simulink model "filtro2_fir_sim_r2015a"  (Simulink 8.5)
settings: Solver=FixedStepDiscrete  SolverMode=SingleTasking  StartTime=0.0  StopTime=1  RelTol=1e-3
values from neighbouring files (symbols this model uses):
  fa = 10000    [filtro2_fir.m]    (also in filtro2_iir.m)
undefined symbols (not defined in the file or in its folder): Ta
libraries: dspsrcs4 x4, dsparch4 x1
settings Model: Creator=vini  LastModifiedBy=vinicius.ls  CovMetricSettings=dwe  CovHtmlReporting=off  covSaveCumulativeToWorkspaceVar=off  CovSaveSingleToWorkspaceVar=off  CovExternalEMLEnable=on
settings DataIOCC: LimitDataPoints=off  SaveFormat=Dataset  SignalLoggingSaveFormat=Dataset
settings OptimizationCC: BlockReduction=off  ConditionallyExecuteInputs=off  InlineParams=on  ExpressionDepthLimit=128
settings DebuggingCC: AlgebraicLoopMsg=error  UnderspecifiedInitializationDetection=Simplified  MergeDetectMultiDrivingBlocksExec=error  FcnCallInpInsideContextMsg=EnableAllAsError  StateNameClashWarn=none  SFUnexpectedBacktrackingDiag=error  SFNoUnconditionalDefaultTransitionDiag=error
settings HardwareCC: ProdHWDeviceType=ASIC/FPGA->ASIC/FPGA  ProdEqTarget=off
settings ModelReferenceCC: PropagateSignalLabelsOutOfModel=on
settings SFSimCC: SimUseLocalCustomCode=on
settings RTWCC: RTWUseLocalCustomCode=on
settings GRTTargetCC: TargetLangStandard=C99 (ISO)  GeneratePreprocessorConditionals=Use local settings  CombineOutputUpdateFcns=on  GRTInterface=off

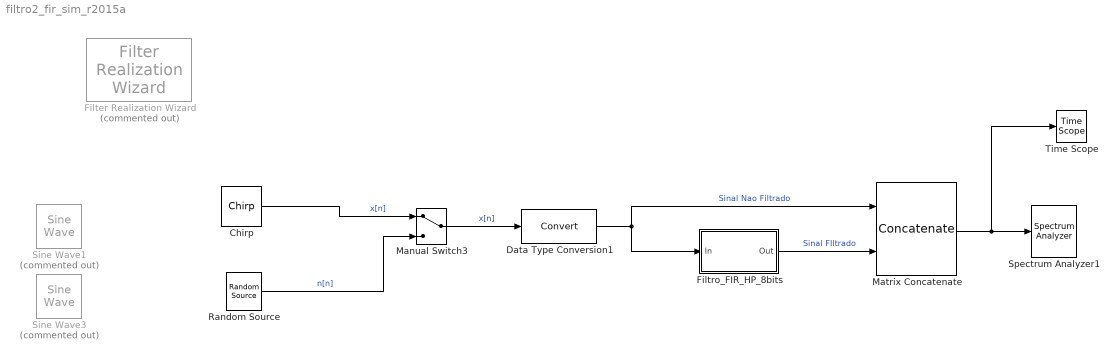
== system filtro2_fir_sim_r2015a ==
  Chirp : dspsrcs4/Chirp  sweep=Linear  mode=Unidirectional  f0=0  f1=fa/2  t1=1  Tsweep=1  phase=0  Ts=Ta  spf=spf  datatype=Double
  Data Type Conversion1 : DataTypeConversion
  Filter Realization Wizard : dsparch4/Filter Realization Wizard  Commented=on
  Filtro_FIR_HP_8bits : Subsystem  Tag=BlockMethodSubSystem
  Manual Switch3 : ManualSwitch
  Matrix Concatenate : Concatenate  Mode=Multidimensional array  ConcatenateDimension=2
  Random Source : dspsrcs4/Random Source  SrcType=Uniform  NormMethod=Ziggurat  CltLength=12  MinVal=-1  MaxVal=1  MeanVal=0  VarVal=1  RepMode=Not repeatable  rawSeed=1  IsInherit=off  SampMode=Discrete  SampTime=Ta  SampFrame=spf  DataType=Single  OutComplex=Real
  Sine Wave1 : dspsrcs4/Sine Wave  Commented=on  Amplitude=1  Frequency=100  Phase=0  SampleMode=Discrete  OutComplex=Real  CompMethod=Trigonometric fcn  TableSize=Speed  SampleTime=1/8000  SamplesPerFrame=1  ResetState=Restart at time zero  dataType=double  wordLen=16  udDataType=sfix(16)  fracBitsMode=Best precision  numFracBits=15  OutDataTypeStr=double  LastOutDataTypeStr=double
  Sine Wave3 : dspsrcs4/Sine Wave  Commented=on  Amplitude=1  Frequency=100  Phase=0  SampleMode=Discrete  OutComplex=Real  CompMethod=Trigonometric fcn  TableSize=Speed  SampleTime=1/8000  SamplesPerFrame=1  ResetState=Restart at time zero  dataType=double  wordLen=16  udDataType=sfix(16)  fracBitsMode=Best precision  numFracBits=15  OutDataTypeStr=double  LastOutDataTypeStr=double
  Spectrum Analyzer1 : SpectrumAnalyzer
  Time Scope : TimeScope  DefaultConfigurationName=spbscopes.TimeScopeBlockCfg
  wires:
  Data Type Conversion1/1 -> Filtro_FIR_HP_8bits/1(In), Matrix Concatenate/1  "Sinal Nao Filtrado"
  Matrix Concatenate/1 -> Time Scope/1, Spectrum Analyzer1/1
  Filtro_FIR_HP_8bits/1(Out) -> Matrix Concatenate/2  "Sinal FIltrado"
  Manual Switch3/1 -> Data Type Conversion1/1  "x[n]"
  Random Source/1 -> Manual Switch3/2  "n[n]"
  Chirp/1 -> Manual Switch3/1  "x[n]"

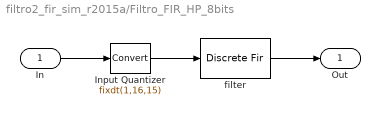
== system filtro2_fir_sim_r2015a/Filtro_FIR_HP_8bits ==
  In : Inport
  Input Quantizer : DataTypeConversion  OutDataTypeStr=fixdt(1,16,15)  RndMeth=Round  SaturateOnIntegerOverflow=on
  filter : DiscreteFir  FilterStructure=Direct form symmetric  Coefficients=[-0.00532709506172761044 0.00150016559407488014 0.00628495279823278012 -0.00636828988327803585 -0.00403452349221034706 0.0111906482400220622 -0.00231967061384724497 -0.0130613282623932899 0.01189990154197915 0.00894421000991611065 -0.0216421575545340458 0.0030362156599829525 0.0265962407774834042 -0.0224925554974460436 -0.0206671663559229203 0.0463858207415749138 -0.00352514866909382297 -0.0696283973383888116 0.0620411228742990054 0.0865544797646948944 -0.292552788167892264 0.389496680318399457 -0.292552788167892264 0.0865544797646948944 0.0620411228742990054 -0.0696283973383888116 -0.00352514866909382297 0.0463858207415749138 -0.0206671663559229203 -0.0224925554974460436 0.0265962407774834042 0.0030362156599829525 -0.0216421575545340458 0.00894421000991611065 0.01189990154197915 -0.0130613282623932899 -0.00231967061384724497 0.0111906482400220622 -0.00403452349221034706 -0.00636828988327803585 0.00628495279823278012 0.00150016559407488014 -0.00532709506172761044]  TapSumDataTypeStr=fixdt(true,17,15)  CoefDataTypeStr=fixdt(true,8,8)  ProductDataTypeStr=fixdt(true,24,23)  AccumDataTypeStr=fixdt(true,25,23)  OutDataTypeStr=fixdt(true,25,23)  RndMeth=Convergent
  Out : Outport
  wires:
  In/1 -> Input Quantizer/1
  Input Quantizer/1 -> filter/1
  filter/1 -> Out/1
